simulink model "winter_simulink"  (R2022b)
settings: Solver=FixedStepAuto  StartTime=0.0  StopTime=300  FixedStep=sample_time/10  RelTol=1e-3
undefined symbols (not defined in the file): cP_vs_lambda, generator, omega_r, rho, rotor, sample_time
settings Model: Creator=Niccolò  LastModifiedBy=user
settings ModelReferenceCC: EnableRefExpFcnMdlSchedulingChecks=on

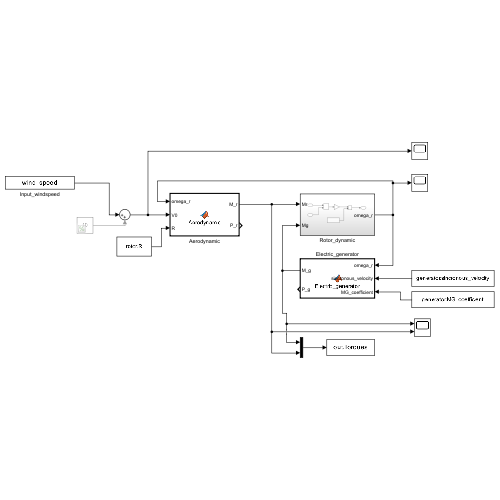
[thumbnail: Simulink's stored preview of the top-level diagram]
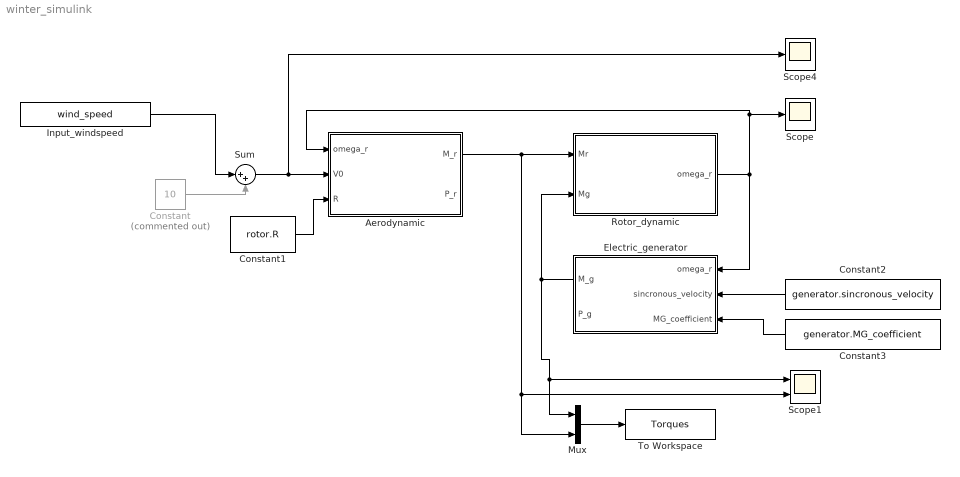
== system winter_simulink ==
  Aerodynamic : MATLAB Function  TreatAsAtomicUnit=on
  Constant : Constant  Commented=on  Value=10
  Constant1 : Constant  Value=rotor.R
  Constant2 : Constant  Value=generator.sincronous_velocity
  Constant3 : Constant  Value=generator.MG_coefficient
  Electric_generator : MATLAB Function  TreatAsAtomicUnit=on
  Input_windspeed : FromWorkspace  VariableName=wind_speed  SampleTime=sample_time
  Mux : Mux  Inputs=2
  Rotor_dynamic : Subsystem
  Scope : Scope
  Scope1 : Scope  NumInputPorts=2
  Scope4 : Scope
  Sum : Sum  Inputs=|++
  To Workspace : ToWorkspace  VariableName=Torques  SampleTime=-1
  wires:
  Aerodynamic/1(M_r) -> Rotor_dynamic/1(Mr), Mux/2, Scope1/2
  Electric_generator/1(M_g) -> Rotor_dynamic/2(Mg), Mux/1, Scope1/1
  Input_windspeed/1 -> Sum/1
  Constant/1 -> Sum/2
  Sum/1 -> Scope4/1, Aerodynamic/2(V0)
  Rotor_dynamic/1(omega_r) -> Aerodynamic/1(omega_r), Scope/1, Electric_generator/1(omega_r)
  Mux/1 -> To Workspace/1
  Constant1/1 -> Aerodynamic/3(R)
  Constant2/1 -> Electric_generator/2(sincronous_velocity)
  Constant3/1 -> Electric_generator/3(MG_coefficient)

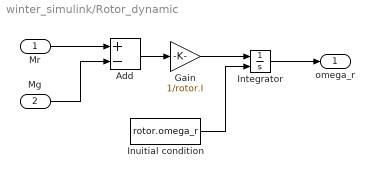
== system winter_simulink/Rotor_dynamic ==
  Mr : Inport
  Mg : Inport  Port=2
  Add : Sum  Inputs=+-
  Gain : Gain  Gain=1/rotor.I
  Integrator : Integrator  InitialConditionSource=external  InitialCondition=omega_r
  Inuitial condition : Constant  Value=rotor.omega_r
  omega_r : Outport
  wires:
  Add/1 -> Gain/1
  Gain/1 -> Integrator/1
  Mr/1 -> Add/1
  Integrator/1 -> omega_r/1
  Mg/1 -> Add/2
  Inuitial condition/1 -> Integrator/2

== matlab function winter_simulink/Aerodynamic ==
  data: omega_r input; V0 input; M_r output; P_r output; rho parameter; cP_vs_lambda parameter; R input
function [M_r, P_r] = Aerodynamic(omega_r, V0, rho, cP_vs_lambda, R) 

lambda = omega_r*R/V0; % tip speed ratio
cP = interp1(cP_vs_lambda(:,1), cP_vs_lambda(:,2), lambda); % interpolate the table

P_r = 0.5*rho*V0^3*pi*R^2*cP; % rotor power [W]
M_r = P_r/omega_r; % rotor torque [Nm]

== matlab function winter_simulink/Electric_generator ==
  data: omega_r input; M_g output; P_g output; sincronous_velocity input; MG_coefficient input
function [M_g, P_g] = Electric_generator(omega_r, sincronous_velocity, ... 
MG_coefficient)

if omega_r < sincronous_velocity
  M_g = 0;
else
  M_g = MG_coefficient*(omega_r - sincronous_velocity);
end

P_g = M_g*omega_r;
